simulink library "fsw_telemetry_bus"  (R2018b)
settings: Solver=VariableStepAuto  StartTime=0.0  StopTime=10.0  RelTol=1e-3
undefined symbols (not defined in the file): fswParams
settings Model: Creator=colem  LastModifiedBy=Taylor

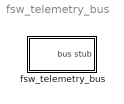
== system fsw_telemetry_bus ==
  fsw_telemetry_bus : Subsystem

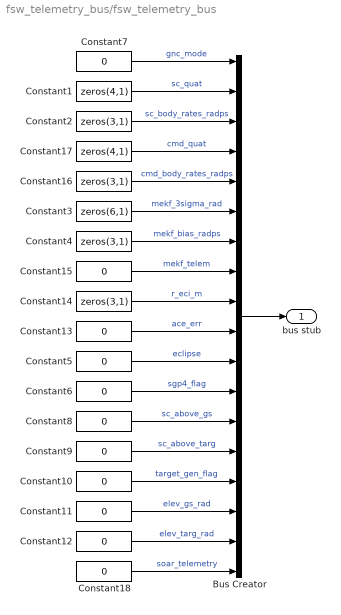
== system fsw_telemetry_bus/fsw_telemetry_bus ==
  Bus Creator : BusCreator  Inputs=18  OutDataTypeStr=Bus: fsw_telemetry
  Constant1 : Constant  Value=zeros(4,1)  OutDataTypeStr=double  SampleTime=fswParams.sample_time_s
  Constant{6..7,10,15} (4 alike) : Constant  Value=0  OutDataTypeStr=uint8  SampleTime=fswParams.sample_time_s
  Constant11 : Constant  Value=0  OutDataTypeStr=double  SampleTime=fswParams.sample_time_s
  Constant12 : Constant  Value=0  OutDataTypeStr=double  SampleTime=fswParams.sample_time_s
  Constant13 : Constant  Value=0  OutDataTypeStr=double  SampleTime=fswParams.sample_time_s
  Constant{2,4,14,16} (4 alike) : Constant  Value=zeros(3,1)  OutDataTypeStr=double  SampleTime=fswParams.sample_time_s
  Constant17 : Constant  Value=zeros(4,1)  OutDataTypeStr=double  SampleTime=fswParams.sample_time_s
  Constant18 : Constant  Value=0  OutDataTypeStr=Bus: soar_telemetry  SampleTime=fswParams.sample_time_s
  Constant3 : Constant  Value=zeros(6,1)  OutDataTypeStr=double  SampleTime=fswParams.sample_time_s
  Constant5 : Constant  Value=0  OutDataTypeStr=boolean  SampleTime=fswParams.sample_time_s
  Constant8 : Constant  Value=0  OutDataTypeStr=boolean  SampleTime=fswParams.sample_time_s
  Constant9 : Constant  Value=0  OutDataTypeStr=boolean  SampleTime=fswParams.sample_time_s
  bus stub : Outport  OutDataTypeStr=Bus: fsw_telemetry
  wires:
  Bus Creator/1 -> bus stub/1
  Constant7/1 -> Bus Creator/1  "gnc_mode"
  Constant1/1 -> Bus Creator/2  "sc_quat"
  Constant2/1 -> Bus Creator/3  "sc_body_rates_radps"
  Constant3/1 -> Bus Creator/6  "mekf_3sigma_rad"
  Constant4/1 -> Bus Creator/7  "mekf_bias_radps"
  Constant12/1 -> Bus Creator/17  "elev_targ_rad"
  Constant11/1 -> Bus Creator/16  "elev_gs_rad"
  Constant10/1 -> Bus Creator/15  "target_gen_flag"
  Constant9/1 -> Bus Creator/14  "sc_above_targ"
  Constant8/1 -> Bus Creator/13  "sc_above_gs"
  Constant6/1 -> Bus Creator/12  "sgp4_flag"
  Constant5/1 -> Bus Creator/11  "eclipse"
  Constant13/1 -> Bus Creator/10  "ace_err"
  Constant14/1 -> Bus Creator/9  "r_eci_m"
  Constant15/1 -> Bus Creator/8  "mekf_telem"
  Constant16/1 -> Bus Creator/5  "cmd_body_rates_radps"
  Constant17/1 -> Bus Creator/4  "cmd_quat"
  Constant18/1 -> Bus Creator/18  "soar_telemetry"
